simulink model "HANcoder_E407_GTSync_v5"  (R2018b)
settings: Solver=FixedStepDiscrete  StartTime=0.0  StopTime=1  FixedStep=0.01  RelTol=1e-3
PreLoadFcn:
  | librarySetup
  | eval([bdroot,'_startup']) %Calling [modelName]_startup.m
values from neighbouring files (symbols this model uses):
  basic_cycle_duration = TM_Reset_Board + COMP_duration    (= 170)    [HANcoder_E407_GTSync_v5_startup.m]
  comm_delay_estimation1 = round(comm_delay_measured*hardware_granularity/frequency_IRQ)    [HANcoder_E407_GTSync_v5_startup.m]
  comm_delay_estimation2 = round(comm_delay_measured*hardware_granularity/frequency_IRQ)    [HANcoder_E407_GTSync_v5_startup.m]
  COMM_Period = 25    [HANcoder_E407_GTSync_v5_startup.m]
  COMM_Phase1 = floor(COMM_Period/5)    [HANcoder_E407_GTSync_v5_startup.m]
  COMM_Phase2 = floor(4*COMM_Period/5)    [HANcoder_E407_GTSync_v5_startup.m]
  frequency_IRQ = 100    [HANcoder_E407_GTSync_v5_startup.m]
  HANtuneOverride = Simulink.Parameter    [HANcoder_E407_GTSync_v5_startup.m]
  idle_time_init = basic_cycle_duration*matrix_rows    (= 340)    [HANcoder_E407_GTSync_v5_startup.m]
  LED_ticks_toggle = 10000    [HANcoder_E407_GTSync_v5_startup.m]
  Master_Role = 1    [HANcoder_E407_GTSync_v5_startup.m]
  matrix_rows = 2    [HANcoder_E407_GTSync_v5_startup.m]
  MEX_Flag = 0    [HANcoder_E407_GTSync_v5_startup.m]
  Slave_Role = 2    [HANcoder_E407_GTSync_v5_startup.m]
  Sync_ID = 1    [HANcoder_E407_GTSync_v5_startup.m]
  TM_Check_Sync = TM_COMM_Sync   + COMM_duration    (= 30)    [HANcoder_E407_GTSync_v5_startup.m]
  TM_Check_TOuts = TM_Count_Vote3 + COMP_duration    (= 150)    [HANcoder_E407_GTSync_v5_startup.m]
  TM_Check_Vote1 = TM_COMM_Vote1  + COMM_duration    (= 70)    [HANcoder_E407_GTSync_v5_startup.m]
  TM_Check_Vote2 = TM_COMM_Vote2  + COMM_duration    (= 105)    [HANcoder_E407_GTSync_v5_startup.m]
  TM_Check_Vote3 = TM_COMM_Vote3  + COMM_duration    (= 140)    [HANcoder_E407_GTSync_v5_startup.m]
  TM_COMM_Sync = basic_cycle_start    (= 5)    [HANcoder_E407_GTSync_v5_startup.m]
  TM_COMM_Vote1 = TM_Vote_Dec    + COMP_duration    (= 45)    [HANcoder_E407_GTSync_v5_startup.m]
  TM_COMM_Vote2 = TM_Count_Vote1 + COMP_duration    (= 80)    [HANcoder_E407_GTSync_v5_startup.m]
  TM_COMM_Vote3 = TM_Count_Vote2 + COMP_duration    (= 115)    [HANcoder_E407_GTSync_v5_startup.m]
  TM_Count_Vote1 = TM_Check_Vote1 + COMP_duration    (= 75)    [HANcoder_E407_GTSync_v5_startup.m]
  TM_Count_Vote2 = TM_Check_Vote2 + COMP_duration    (= 110)    [HANcoder_E407_GTSync_v5_startup.m]
  TM_Count_Vote3 = TM_Check_Vote3 + COMP_duration    (= 145)    [HANcoder_E407_GTSync_v5_startup.m]
  TM_New_Master = TM_Check_TOuts + COMP_duration    (= 155)    [HANcoder_E407_GTSync_v5_startup.m]
  TM_Reset_Board = TM_Reset_Var   + COMP_duration    (= 165)    [HANcoder_E407_GTSync_v5_startup.m]
  TM_Reset_Var = TM_New_Master  + COMP_duration    (= 160)    [HANcoder_E407_GTSync_v5_startup.m]
  TM_Update_LT = TM_Check_Sync  + COMP_duration    (= 35)    [HANcoder_E407_GTSync_v5_startup.m]
  TM_Vote_Dec = TM_Update_LT   + COMP_duration    (= 40)    [HANcoder_E407_GTSync_v5_startup.m]
  Toggle_Flag = 1    [HANcoder_E407_GTSync_v5_startup.m]
  Vote1_ID = 12    [HANcoder_E407_GTSync_v5_startup.m]
  Vote2_ID = 22    [HANcoder_E407_GTSync_v5_startup.m]
  Vote3_ID = 32    [HANcoder_E407_GTSync_v5_startup.m]
undefined symbols (not defined in the file or in its folder): A0, A1, A2, A3, CON2
libraries: HANcoder_STM32_Target x25, hdlsllib x21, simulink x3, simulink_extras x1
(part 4 of 7)

== system HANcoder_E407_GTSync_v5/HANcoder STM32 Target - E407-STM32 algorithm/Global Ticks Increment/CAN Management/Matrix Cycle Manager/Matrix_Cycle_Observation_DEBUG ==
  Data Store Read : DataStoreRead  DataStoreName=Master_ID
  Data Store Read1 : DataStoreRead  DataStoreName=Role_ID
  Data Store Read10 : DataStoreRead  DataStoreName=time_difference_vote3
  Data Store Read11 : DataStoreRead  DataStoreName=sync_processed
  Data Store Read12 : DataStoreRead  DataStoreName=Rx_State_CAN1
  Data Store Read13 : DataStoreRead  DataStoreName=New_Msg_Ready_CAN1
  Data Store Read2 : DataStoreRead  DataStoreName=received_LT  DataStoreElements=received_LT.Local_Time_Board_1#received_LT.Local_Time_Board_2#received_LT.Local_Time_Board_3
  Data Store Read3 : DataStoreRead  DataStoreName=votes  DataStoreElements=votes.First_Board#votes.Second_Board#votes.Third_Board
  Data Store Read4 : DataStoreRead  DataStoreName=Board1_error_counter
  Data Store Read5 : DataStoreRead  DataStoreName=Board2_error_counter
  Data Store Read6 : DataStoreRead  DataStoreName=Board3_error_counter
  Data Store Read7 : DataStoreRead  DataStoreName=time_difference_sync
  Data Store Read8 : DataStoreRead  DataStoreName=time_difference_vote1
  Data Store Read9 : DataStoreRead  DataStoreName=time_difference_vote2
  Terminator{,1..17} (18 alike) : Terminator
  wires:
  Data Store Read1/1 -> Terminator/1  "Role_ID_DEBUG"
  Data Store Read/1 -> Terminator1/1  "Master_ID_DEBUG"
  Data Store Read2/1 -> Terminator2/1  "received_LT_Board_1_DEBUG"
  Data Store Read2/2 -> Terminator3/1  "received_LT_Board_2_DEBUG"
  Data Store Read2/3 -> Terminator4/1  "received_LT_Board_3_DEBUG"
  Data Store Read3/1 -> Terminator5/1  "votes_Board_1_DEBUG"
  Data Store Read3/2 -> Terminator6/1  "votes_Board_2_DEBUG"
  Data Store Read3/3 -> Terminator7/1  "votes_Board_3_DEBUG"
  Data Store Read4/1 -> Terminator8/1  "Board_1_error_counter_DEBUG"
  Data Store Read5/1 -> Terminator9/1  "Board_2_error_counter_DEBUG"
  Data Store Read6/1 -> Terminator10/1  "Board_3_error_counter_DEBUG"
  Data Store Read7/1 -> Terminator11/1  "time_difference_sync_DEBUG"
  Data Store Read8/1 -> Terminator12/1  "time_difference_vote_1_DEBUG"
  Data Store Read9/1 -> Terminator13/1  "time_difference_vote_2_DEBUG"
  Data Store Read10/1 -> Terminator14/1  "time_difference_vote_3_DEBUG"
  Data Store Read11/1 -> Terminator15/1  "sync_processed_s"
  Data Store Read12/1 -> Terminator16/1  "rx_state_s"
  Data Store Read13/1 -> Terminator17/1  "new_msg_ready_s"

== system HANcoder_E407_GTSync_v5/HANcoder STM32 Target - E407-STM32 algorithm/Global Ticks Increment/CAN1 Recieve/CAN receive/Enabled Subsystem ==
  In1 : Inport
  In2 : Inport  Port=2
  In3 : Inport  Port=3
  In4 : Inport  Port=4
  In5 : Inport  Port=5
  In6 : Inport  Port=6
  In7 : Inport  Port=7
  In8 : Inport  Port=8
  Enable : EnablePort
  Out1 : Outport
  Out2 : Outport  Port=2
  Out3 : Outport  Port=3
  Out4 : Outport  Port=4
  Out5 : Outport  Port=5
  Out6 : Outport  Port=6
  Out7 : Outport  Port=7
  Out8 : Outport  Port=8
  wires:
  In8/1 -> Out8/1
  In7/1 -> Out7/1
  In6/1 -> Out6/1
  In5/1 -> Out5/1
  In4/1 -> Out4/1
  In3/1 -> Out3/1
  In2/1 -> Out2/1
  In1/1 -> Out1/1

== system HANcoder_E407_GTSync_v5/HANcoder STM32 Target - E407-STM32 algorithm/Global Ticks Increment/CAN1 Recieve/RxID_CAN/Sync_ID_CAN ==
  Enable : EnablePort
  CAN receive : Subsystem  Tag=HANcoder_TARGET_STM32_E407  AncestorBlock=HANcoder_STM32_Target/STM32-E407/CAN/CAN/CAN receive  mask(CAN receive){canBus=CAN 1, outputNumber=8, dataType=uint8, byteOrder=off, tsamp=-1}
      mask prompts: canBus "CAN channel"; outputNumber "Output ports"; dataType "Output datatype"; byteOrder "Byte order: Checked = MSB first, unchecked = LSB first."; tsamp "Sample time"
      mask help:
      | Function
      | ==========
      | Receive the newest message from the specified CAN channel.
      |
      | Parameters
      | ==========
      | CAN channel:             The CAN channel to send the message on.
      | Output ports:             The amount of output ports
      | Output datatype:       The datatype of the output ports
      | Byte order:                 Select MSB or LSB first
      | Sample time:              -1 or divisible by base sample time [seconds]
      |
      | Input
      | ==========
      | Port 1:                       CAN ID(uint32) in hexadecimal ie: hex2dec('0a')
      |
      | Output
      | ==========
      | Port 1:                       Checks for new message(int8)
      | Port 2..9                     Message data
      mask init:
      | sfcn_can_receive_mcb(canBus, outputNumber, dataType, byteOrder)
      settings: MoveFcn=drawLogos
      mask Help: web('sfcn_can_receive.html');
      mask TypeOptions canBus: CAN 1 | CAN 2
      mask TypeOptions dataType: int8 | uint8 | int16 | uint16 | int32 | uint32 | boolean
      mask Display:
      | fprintf('Receive on\nCAN %x', canBus);
      | port_label('output', 1, 'new');
      | port_label('input', 1, 'ID');patch([135 141 141],[8 14 2],[1 0 0]);patch([143 143 149],[14 2 8],[0 0 0.35]);
  Constant : Constant  Value=Sync_ID  OutDataTypeStr=uint32
  CAN_new : Outport  OutputWhenDisabled=reset  InitialOutput=0
  Out2 : Outport  Port=2  OutputWhenDisabled=reset  InitialOutput=0
  Out3 : Outport  Port=3  OutputWhenDisabled=reset  InitialOutput=0
  Out4 : Outport  Port=4  OutputWhenDisabled=reset  InitialOutput=0
  Out5 : Outport  Port=5  OutputWhenDisabled=reset  InitialOutput=0
  Out6 : Outport  Port=6  OutputWhenDisabled=reset  InitialOutput=0
  Out7 : Outport  Port=7  OutputWhenDisabled=reset  InitialOutput=0
  Out8 : Outport  Port=8  OutputWhenDisabled=reset  InitialOutput=0
  Out9 : Outport  Port=9  OutputWhenDisabled=reset  InitialOutput=0
  wires:
  CAN receive/1(Out1) -> CAN_new/1
  CAN receive/8(Out8) -> Out8/1
  CAN receive/3(Out3) -> Out3/1
  Constant/1 -> CAN receive/1(In1)
  CAN receive/2(Out2) -> Out2/1
  CAN receive/6(Out6) -> Out6/1
  CAN receive/7(Out7) -> Out7/1
  CAN receive/4(Out4) -> Out4/1
  CAN receive/5(Out5) -> Out5/1
  CAN receive/9(Out9) -> Out9/1

== system HANcoder_E407_GTSync_v5/HANcoder STM32 Target - E407-STM32 algorithm/Global Ticks Increment/CAN1 Recieve/RxID_CAN/Vote1_ID_CAN ==
  Enable : EnablePort
  CAN receive : Subsystem  Tag=HANcoder_TARGET_STM32_E407  AncestorBlock=HANcoder_STM32_Target/STM32-E407/CAN/CAN/CAN receive  mask(CAN receive){canBus=CAN 1, outputNumber=8, dataType=uint8, byteOrder=off, tsamp=-1}
      mask prompts: canBus "CAN channel"; outputNumber "Output ports"; dataType "Output datatype"; byteOrder "Byte order: Checked = MSB first, unchecked = LSB first."; tsamp "Sample time"
      mask help:
      | Function
      | ==========
      | Receive the newest message from the specified CAN channel.
      |
      | Parameters
      | ==========
      | CAN channel:             The CAN channel to send the message on.
      | Output ports:             The amount of output ports
      | Output datatype:       The datatype of the output ports
      | Byte order:                 Select MSB or LSB first
      | Sample time:              -1 or divisible by base sample time [seconds]
      |
      | Input
      | ==========
      | Port 1:                       CAN ID(uint32) in hexadecimal ie: hex2dec('0a')
      |
      | Output
      | ==========
      | Port 1:                       Checks for new message(int8)
      | Port 2..9                     Message data
      mask init:
      | sfcn_can_receive_mcb(canBus, outputNumber, dataType, byteOrder)
      settings: MoveFcn=drawLogos
      mask Help: web('sfcn_can_receive.html');
      mask TypeOptions canBus: CAN 1 | CAN 2
      mask TypeOptions dataType: int8 | uint8 | int16 | uint16 | int32 | uint32 | boolean
      mask Display:
      | fprintf('Receive on\nCAN %x', canBus);
      | port_label('output', 1, 'new');
      | port_label('input', 1, 'ID');patch([135 141 141],[8 14 2],[1 0 0]);patch([143 143 149],[14 2 8],[0 0 0.35]);
  Constant : Constant  Value=Vote1_ID  OutDataTypeStr=uint32
  CAN_new : Outport  OutputWhenDisabled=reset  InitialOutput=0
  Out2 : Outport  Port=2  OutputWhenDisabled=reset  InitialOutput=0
  Out3 : Outport  Port=3  OutputWhenDisabled=reset  InitialOutput=0
  Out4 : Outport  Port=4  OutputWhenDisabled=reset  InitialOutput=0
  Out5 : Outport  Port=5  OutputWhenDisabled=reset  InitialOutput=0
  Out6 : Outport  Port=6  OutputWhenDisabled=reset  InitialOutput=0
  Out7 : Outport  Port=7  OutputWhenDisabled=reset  InitialOutput=0
  Out8 : Outport  Port=8  OutputWhenDisabled=reset  InitialOutput=0
  Out9 : Outport  Port=9  OutputWhenDisabled=reset  InitialOutput=0
  wires:
  CAN receive/9(Out9) -> Out9/1
  CAN receive/5(Out5) -> Out5/1
  CAN receive/4(Out4) -> Out4/1
  CAN receive/7(Out7) -> Out7/1
  CAN receive/6(Out6) -> Out6/1
  CAN receive/2(Out2) -> Out2/1
  Constant/1 -> CAN receive/1(In1)
  CAN receive/3(Out3) -> Out3/1
  CAN receive/8(Out8) -> Out8/1
  CAN receive/1(Out1) -> CAN_new/1

== system HANcoder_E407_GTSync_v5/HANcoder STM32 Target - E407-STM32 algorithm/Global Ticks Increment/CAN1 Recieve/RxID_CAN/Vote2_ID_CAN ==
  Enable : EnablePort
  CAN receive : Subsystem  Tag=HANcoder_TARGET_STM32_E407  AncestorBlock=HANcoder_STM32_Target/STM32-E407/CAN/CAN/CAN receive  mask(CAN receive){canBus=CAN 1, outputNumber=8, dataType=uint8, byteOrder=off, tsamp=-1}
      mask prompts: canBus "CAN channel"; outputNumber "Output ports"; dataType "Output datatype"; byteOrder "Byte order: Checked = MSB first, unchecked = LSB first."; tsamp "Sample time"
      mask help:
      | Function
      | ==========
      | Receive the newest message from the specified CAN channel.
      |
      | Parameters
      | ==========
      | CAN channel:             The CAN channel to send the message on.
      | Output ports:             The amount of output ports
      | Output datatype:       The datatype of the output ports
      | Byte order:                 Select MSB or LSB first
      | Sample time:              -1 or divisible by base sample time [seconds]
      |
      | Input
      | ==========
      | Port 1:                       CAN ID(uint32) in hexadecimal ie: hex2dec('0a')
      |
      | Output
      | ==========
      | Port 1:                       Checks for new message(int8)
      | Port 2..9                     Message data
      mask init:
      | sfcn_can_receive_mcb(canBus, outputNumber, dataType, byteOrder)
      settings: MoveFcn=drawLogos
      mask Help: web('sfcn_can_receive.html');
      mask TypeOptions canBus: CAN 1 | CAN 2
      mask TypeOptions dataType: int8 | uint8 | int16 | uint16 | int32 | uint32 | boolean
      mask Display:
      | fprintf('Receive on\nCAN %x', canBus);
      | port_label('output', 1, 'new');
      | port_label('input', 1, 'ID');patch([135 141 141],[8 14 2],[1 0 0]);patch([143 143 149],[14 2 8],[0 0 0.35]);
  Constant : Constant  Value=Vote2_ID  OutDataTypeStr=uint32
  CAN_new : Outport  OutputWhenDisabled=reset  InitialOutput=0
  Out2 : Outport  Port=2  OutputWhenDisabled=reset  InitialOutput=0
  Out3 : Outport  Port=3  OutputWhenDisabled=reset  InitialOutput=0
  Out4 : Outport  Port=4  OutputWhenDisabled=reset  InitialOutput=0
  Out5 : Outport  Port=5  OutputWhenDisabled=reset  InitialOutput=0
  Out6 : Outport  Port=6  OutputWhenDisabled=reset  InitialOutput=0
  Out7 : Outport  Port=7  OutputWhenDisabled=reset  InitialOutput=0
  Out8 : Outport  Port=8  OutputWhenDisabled=reset  InitialOutput=0
  Out9 : Outport  Port=9  OutputWhenDisabled=reset  InitialOutput=0
  wires:
  CAN receive/1(Out1) -> CAN_new/1
  CAN receive/8(Out8) -> Out8/1
  CAN receive/3(Out3) -> Out3/1
  Constant/1 -> CAN receive/1(In1)
  CAN receive/2(Out2) -> Out2/1
  CAN receive/6(Out6) -> Out6/1
  CAN receive/7(Out7) -> Out7/1
  CAN receive/4(Out4) -> Out4/1
  CAN receive/5(Out5) -> Out5/1
  CAN receive/9(Out9) -> Out9/1

== system HANcoder_E407_GTSync_v5/HANcoder STM32 Target - E407-STM32 algorithm/Global Ticks Increment/CAN1 Recieve/RxID_CAN/Vote3_ID_CAN ==
  Enable : EnablePort
  CAN receive : Subsystem  Tag=HANcoder_TARGET_STM32_E407  AncestorBlock=HANcoder_STM32_Target/STM32-E407/CAN/CAN/CAN receive  mask(CAN receive){canBus=CAN 1, outputNumber=8, dataType=uint8, byteOrder=off, tsamp=-1}
      mask prompts: canBus "CAN channel"; outputNumber "Output ports"; dataType "Output datatype"; byteOrder "Byte order: Checked = MSB first, unchecked = LSB first."; tsamp "Sample time"
      mask help:
      | Function
      | ==========
      | Receive the newest message from the specified CAN channel.
      |
      | Parameters
      | ==========
      | CAN channel:             The CAN channel to send the message on.
      | Output ports:             The amount of output ports
      | Output datatype:       The datatype of the output ports
      | Byte order:                 Select MSB or LSB first
      | Sample time:              -1 or divisible by base sample time [seconds]
      |
      | Input
      | ==========
      | Port 1:                       CAN ID(uint32) in hexadecimal ie: hex2dec('0a')
      |
      | Output
      | ==========
      | Port 1:                       Checks for new message(int8)
      | Port 2..9                     Message data
      mask init:
      | sfcn_can_receive_mcb(canBus, outputNumber, dataType, byteOrder)
      settings: MoveFcn=drawLogos
      mask Help: web('sfcn_can_receive.html');
      mask TypeOptions canBus: CAN 1 | CAN 2
      mask TypeOptions dataType: int8 | uint8 | int16 | uint16 | int32 | uint32 | boolean
      mask Display:
      | fprintf('Receive on\nCAN %x', canBus);
      | port_label('output', 1, 'new');
      | port_label('input', 1, 'ID');patch([135 141 141],[8 14 2],[1 0 0]);patch([143 143 149],[14 2 8],[0 0 0.35]);
  Constant : Constant  Value=Vote3_ID  OutDataTypeStr=uint32
  CAN_new : Outport  OutputWhenDisabled=reset  InitialOutput=0
  Out2 : Outport  Port=2  OutputWhenDisabled=reset  InitialOutput=0
  Out3 : Outport  Port=3  OutputWhenDisabled=reset  InitialOutput=0
  Out4 : Outport  Port=4  OutputWhenDisabled=reset  InitialOutput=0
  Out5 : Outport  Port=5  OutputWhenDisabled=reset  InitialOutput=0
  Out6 : Outport  Port=6  OutputWhenDisabled=reset  InitialOutput=0
  Out7 : Outport  Port=7  OutputWhenDisabled=reset  InitialOutput=0
  Out8 : Outport  Port=8  OutputWhenDisabled=reset  InitialOutput=0
  Out9 : Outport  Port=9  OutputWhenDisabled=reset  InitialOutput=0
  wires:
  CAN receive/9(Out9) -> Out9/1
  CAN receive/5(Out5) -> Out5/1
  CAN receive/4(Out4) -> Out4/1
  CAN receive/7(Out7) -> Out7/1
  CAN receive/6(Out6) -> Out6/1
  CAN receive/2(Out2) -> Out2/1
  Constant/1 -> CAN receive/1(In1)
  CAN receive/3(Out3) -> Out3/1
  CAN receive/8(Out8) -> Out8/1
  CAN receive/1(Out1) -> CAN_new/1

== system HANcoder_E407_GTSync_v5/HANcoder STM32 Target - E407-STM32 algorithm/Global Ticks Increment/CAN2 Recieve/CAN receive/Enabled Subsystem ==
  In1 : Inport
  In2 : Inport  Port=2
  In3 : Inport  Port=3
  In4 : Inport  Port=4
  In5 : Inport  Port=5
  In6 : Inport  Port=6
  In7 : Inport  Port=7
  In8 : Inport  Port=8
  Enable : EnablePort
  Out1 : Outport
  Out2 : Outport  Port=2
  Out3 : Outport  Port=3
  Out4 : Outport  Port=4
  Out5 : Outport  Port=5
  Out6 : Outport  Port=6
  Out7 : Outport  Port=7
  Out8 : Outport  Port=8
  wires:
  In8/1 -> Out8/1
  In7/1 -> Out7/1
  In6/1 -> Out6/1
  In5/1 -> Out5/1
  In4/1 -> Out4/1
  In3/1 -> Out3/1
  In2/1 -> Out2/1
  In1/1 -> Out1/1

== system HANcoder_E407_GTSync_v5/HANcoder STM32 Target - E407-STM32 algorithm/Global Ticks Increment/CAN2 Recieve/RxID_CAN/Sync_ID_CAN ==
  Enable : EnablePort
  CAN receive : Subsystem  Tag=HANcoder_TARGET_STM32_E407  AncestorBlock=HANcoder_STM32_Target/STM32-E407/CAN/CAN/CAN receive  mask(CAN receive){canBus=CAN 2, outputNumber=8, dataType=uint8, byteOrder=off, tsamp=-1}
      mask prompts: canBus "CAN channel"; outputNumber "Output ports"; dataType "Output datatype"; byteOrder "Byte order: Checked = MSB first, unchecked = LSB first."; tsamp "Sample time"
      mask help:
      | Function
      | ==========
      | Receive the newest message from the specified CAN channel.
      |
      | Parameters
      | ==========
      | CAN channel:             The CAN channel to send the message on.
      | Output ports:             The amount of output ports
      | Output datatype:       The datatype of the output ports
      | Byte order:                 Select MSB or LSB first
      | Sample time:              -1 or divisible by base sample time [seconds]
      |
      | Input
      | ==========
      | Port 1:                       CAN ID(uint32) in hexadecimal ie: hex2dec('0a')
      |
      | Output
      | ==========
      | Port 1:                       Checks for new message(int8)
      | Port 2..9                     Message data
      mask init:
      | sfcn_can_receive_mcb(canBus, outputNumber, dataType, byteOrder)
      settings: MoveFcn=drawLogos
      mask Help: web('sfcn_can_receive.html');
      mask TypeOptions canBus: CAN 1 | CAN 2
      mask TypeOptions dataType: int8 | uint8 | int16 | uint16 | int32 | uint32 | boolean
      mask Display:
      | fprintf('Receive on\nCAN %x', canBus);
      | port_label('output', 1, 'new');
      | port_label('input', 1, 'ID');patch([135 141 141],[8 14 2],[1 0 0]);patch([143 143 149],[14 2 8],[0 0 0.35]);
  Constant : Constant  Value=Sync_ID  OutDataTypeStr=uint32
  CAN_new : Outport  OutputWhenDisabled=reset  InitialOutput=0
  Out2 : Outport  Port=2  OutputWhenDisabled=reset  InitialOutput=0
  Out3 : Outport  Port=3  OutputWhenDisabled=reset  InitialOutput=0
  Out4 : Outport  Port=4  OutputWhenDisabled=reset  InitialOutput=0
  Out5 : Outport  Port=5  OutputWhenDisabled=reset  InitialOutput=0
  Out6 : Outport  Port=6  OutputWhenDisabled=reset  InitialOutput=0
  Out7 : Outport  Port=7  OutputWhenDisabled=reset  InitialOutput=0
  Out8 : Outport  Port=8  OutputWhenDisabled=reset  InitialOutput=0
  Out9 : Outport  Port=9  OutputWhenDisabled=reset  InitialOutput=0
  wires:
  CAN receive/9(Out9) -> Out9/1
  CAN receive/5(Out5) -> Out5/1
  CAN receive/4(Out4) -> Out4/1
  CAN receive/7(Out7) -> Out7/1
  CAN receive/6(Out6) -> Out6/1
  CAN receive/2(Out2) -> Out2/1
  Constant/1 -> CAN receive/1(In1)
  CAN receive/3(Out3) -> Out3/1
  CAN receive/8(Out8) -> Out8/1
  CAN receive/1(Out1) -> CAN_new/1

== system HANcoder_E407_GTSync_v5/HANcoder STM32 Target - E407-STM32 algorithm/Global Ticks Increment/CAN2 Recieve/RxID_CAN/Vote1_ID_CAN ==
  Enable : EnablePort
  CAN receive : Subsystem  Tag=HANcoder_TARGET_STM32_E407  AncestorBlock=HANcoder_STM32_Target/STM32-E407/CAN/CAN/CAN receive  mask(CAN receive){canBus=CAN 2, outputNumber=8, dataType=uint8, byteOrder=off, tsamp=-1}
      mask prompts: canBus "CAN channel"; outputNumber "Output ports"; dataType "Output datatype"; byteOrder "Byte order: Checked = MSB first, unchecked = LSB first."; tsamp "Sample time"
      mask help:
      | Function
      | ==========
      | Receive the newest message from the specified CAN channel.
      |
      | Parameters
      | ==========
      | CAN channel:             The CAN channel to send the message on.
      | Output ports:             The amount of output ports
      | Output datatype:       The datatype of the output ports
      | Byte order:                 Select MSB or LSB first
      | Sample time:              -1 or divisible by base sample time [seconds]
      |
      | Input
      | ==========
      | Port 1:                       CAN ID(uint32) in hexadecimal ie: hex2dec('0a')
      |
      | Output
      | ==========
      | Port 1:                       Checks for new message(int8)
      | Port 2..9                     Message data
      mask init:
      | sfcn_can_receive_mcb(canBus, outputNumber, dataType, byteOrder)
      settings: MoveFcn=drawLogos
      mask Help: web('sfcn_can_receive.html');
      mask TypeOptions canBus: CAN 1 | CAN 2
      mask TypeOptions dataType: int8 | uint8 | int16 | uint16 | int32 | uint32 | boolean
      mask Display:
      | fprintf('Receive on\nCAN %x', canBus);
      | port_label('output', 1, 'new');
      | port_label('input', 1, 'ID');patch([135 141 141],[8 14 2],[1 0 0]);patch([143 143 149],[14 2 8],[0 0 0.35]);
  Constant : Constant  Value=Vote1_ID  OutDataTypeStr=uint32
  CAN_new : Outport  OutputWhenDisabled=reset  InitialOutput=0
  Out2 : Outport  Port=2  OutputWhenDisabled=reset  InitialOutput=0
  Out3 : Outport  Port=3  OutputWhenDisabled=reset  InitialOutput=0
  Out4 : Outport  Port=4  OutputWhenDisabled=reset  InitialOutput=0
  Out5 : Outport  Port=5  OutputWhenDisabled=reset  InitialOutput=0
  Out6 : Outport  Port=6  OutputWhenDisabled=reset  InitialOutput=0
  Out7 : Outport  Port=7  OutputWhenDisabled=reset  InitialOutput=0
  Out8 : Outport  Port=8  OutputWhenDisabled=reset  InitialOutput=0
  Out9 : Outport  Port=9  OutputWhenDisabled=reset  InitialOutput=0
  wires:
  CAN receive/1(Out1) -> CAN_new/1
  CAN receive/8(Out8) -> Out8/1
  CAN receive/3(Out3) -> Out3/1
  Constant/1 -> CAN receive/1(In1)
  CAN receive/2(Out2) -> Out2/1
  CAN receive/6(Out6) -> Out6/1
  CAN receive/7(Out7) -> Out7/1
  CAN receive/4(Out4) -> Out4/1
  CAN receive/5(Out5) -> Out5/1
  CAN receive/9(Out9) -> Out9/1

== system HANcoder_E407_GTSync_v5/HANcoder STM32 Target - E407-STM32 algorithm/Global Ticks Increment/CAN2 Recieve/RxID_CAN/Vote2_ID_CAN ==
  Enable : EnablePort
  CAN receive : Subsystem  Tag=HANcoder_TARGET_STM32_E407  AncestorBlock=HANcoder_STM32_Target/STM32-E407/CAN/CAN/CAN receive  mask(CAN receive){canBus=CAN 2, outputNumber=8, dataType=uint8, byteOrder=off, tsamp=-1}
      mask prompts: canBus "CAN channel"; outputNumber "Output ports"; dataType "Output datatype"; byteOrder "Byte order: Checked = MSB first, unchecked = LSB first."; tsamp "Sample time"
      mask help:
      | Function
      | ==========
      | Receive the newest message from the specified CAN channel.
      |
      | Parameters
      | ==========
      | CAN channel:             The CAN channel to send the message on.
      | Output ports:             The amount of output ports
      | Output datatype:       The datatype of the output ports
      | Byte order:                 Select MSB or LSB first
      | Sample time:              -1 or divisible by base sample time [seconds]
      |
      | Input
      | ==========
      | Port 1:                       CAN ID(uint32) in hexadecimal ie: hex2dec('0a')
      |
      | Output
      | ==========
      | Port 1:                       Checks for new message(int8)
      | Port 2..9                     Message data
      mask init:
      | sfcn_can_receive_mcb(canBus, outputNumber, dataType, byteOrder)
      settings: MoveFcn=drawLogos
      mask Help: web('sfcn_can_receive.html');
      mask TypeOptions canBus: CAN 1 | CAN 2
      mask TypeOptions dataType: int8 | uint8 | int16 | uint16 | int32 | uint32 | boolean
      mask Display:
      | fprintf('Receive on\nCAN %x', canBus);
      | port_label('output', 1, 'new');
      | port_label('input', 1, 'ID');patch([135 141 141],[8 14 2],[1 0 0]);patch([143 143 149],[14 2 8],[0 0 0.35]);
  Constant : Constant  Value=Vote2_ID  OutDataTypeStr=uint32
  CAN_new : Outport  OutputWhenDisabled=reset  InitialOutput=0
  Out2 : Outport  Port=2  OutputWhenDisabled=reset  InitialOutput=0
  Out3 : Outport  Port=3  OutputWhenDisabled=reset  InitialOutput=0
  Out4 : Outport  Port=4  OutputWhenDisabled=reset  InitialOutput=0
  Out5 : Outport  Port=5  OutputWhenDisabled=reset  InitialOutput=0
  Out6 : Outport  Port=6  OutputWhenDisabled=reset  InitialOutput=0
  Out7 : Outport  Port=7  OutputWhenDisabled=reset  InitialOutput=0
  Out8 : Outport  Port=8  OutputWhenDisabled=reset  InitialOutput=0
  Out9 : Outport  Port=9  OutputWhenDisabled=reset  InitialOutput=0
  wires:
  CAN receive/9(Out9) -> Out9/1
  CAN receive/5(Out5) -> Out5/1
  CAN receive/4(Out4) -> Out4/1
  CAN receive/7(Out7) -> Out7/1
  CAN receive/6(Out6) -> Out6/1
  CAN receive/2(Out2) -> Out2/1
  Constant/1 -> CAN receive/1(In1)
  CAN receive/3(Out3) -> Out3/1
  CAN receive/8(Out8) -> Out8/1
  CAN receive/1(Out1) -> CAN_new/1

== system HANcoder_E407_GTSync_v5/HANcoder STM32 Target - E407-STM32 algorithm/Global Ticks Increment/CAN2 Recieve/RxID_CAN/Vote3_ID_CAN ==
  Enable : EnablePort
  CAN receive : Subsystem  Tag=HANcoder_TARGET_STM32_E407  AncestorBlock=HANcoder_STM32_Target/STM32-E407/CAN/CAN/CAN receive  mask(CAN receive){canBus=CAN 2, outputNumber=8, dataType=uint8, byteOrder=off, tsamp=-1}
      mask prompts: canBus "CAN channel"; outputNumber "Output ports"; dataType "Output datatype"; byteOrder "Byte order: Checked = MSB first, unchecked = LSB first."; tsamp "Sample time"
      mask help:
      | Function
      | ==========
      | Receive the newest message from the specified CAN channel.
      |
      | Parameters
      | ==========
      | CAN channel:             The CAN channel to send the message on.
      | Output ports:             The amount of output ports
      | Output datatype:       The datatype of the output ports
      | Byte order:                 Select MSB or LSB first
      | Sample time:              -1 or divisible by base sample time [seconds]
      |
      | Input
      | ==========
      | Port 1:                       CAN ID(uint32) in hexadecimal ie: hex2dec('0a')
      |
      | Output
      | ==========
      | Port 1:                       Checks for new message(int8)
      | Port 2..9                     Message data
      mask init:
      | sfcn_can_receive_mcb(canBus, outputNumber, dataType, byteOrder)
      settings: MoveFcn=drawLogos
      mask Help: web('sfcn_can_receive.html');
      mask TypeOptions canBus: CAN 1 | CAN 2
      mask TypeOptions dataType: int8 | uint8 | int16 | uint16 | int32 | uint32 | boolean
      mask Display:
      | fprintf('Receive on\nCAN %x', canBus);
      | port_label('output', 1, 'new');
      | port_label('input', 1, 'ID');patch([135 141 141],[8 14 2],[1 0 0]);patch([143 143 149],[14 2 8],[0 0 0.35]);
  Constant : Constant  Value=Vote3_ID  OutDataTypeStr=uint32
  CAN_new : Outport  OutputWhenDisabled=reset  InitialOutput=0
  Out2 : Outport  Port=2  OutputWhenDisabled=reset  InitialOutput=0
  Out3 : Outport  Port=3  OutputWhenDisabled=reset  InitialOutput=0
  Out4 : Outport  Port=4  OutputWhenDisabled=reset  InitialOutput=0
  Out5 : Outport  Port=5  OutputWhenDisabled=reset  InitialOutput=0
  Out6 : Outport  Port=6  OutputWhenDisabled=reset  InitialOutput=0
  Out7 : Outport  Port=7  OutputWhenDisabled=reset  InitialOutput=0
  Out8 : Outport  Port=8  OutputWhenDisabled=reset  InitialOutput=0
  Out9 : Outport  Port=9  OutputWhenDisabled=reset  InitialOutput=0
  wires:
  CAN receive/1(Out1) -> CAN_new/1
  CAN receive/8(Out8) -> Out8/1
  CAN receive/3(Out3) -> Out3/1
  Constant/1 -> CAN receive/1(In1)
  CAN receive/2(Out2) -> Out2/1
  CAN receive/6(Out6) -> Out6/1
  CAN receive/7(Out7) -> Out7/1
  CAN receive/4(Out4) -> Out4/1
  CAN receive/5(Out5) -> Out5/1
  CAN receive/9(Out9) -> Out9/1

== system HANcoder_E407_GTSync_v5/HANcoder STM32 Target - E407-STM32 algorithm/Global Ticks Increment/CAN Management/Initialization/Delay/Initializaton_Observation_DEBUG ==
  Data Store Read : DataStoreRead  DataStoreName=Initialization_flag
  Data Store Read1 : DataStoreRead  DataStoreName=Delay_Counter
  Data Store Read2 : DataStoreRead  DataStoreName=New_Msg_Ready_CAN1
  Data Store Read3 : DataStoreRead  DataStoreName=Initialization_Timeout
  Data Store Read5 : DataStoreRead  DataStoreName=basic_cycle_count
  Terminator{,1..3,5} (5 alike) : Terminator
  wires:
  Data Store Read3/1 -> Terminator3/1  "initialization_timeout_DEBUG"
  Data Store Read1/1 -> Terminator1/1  "delay_counter_DEBUG"
  Data Store Read/1 -> Terminator/1  "initialization_flag_DEBUG"
  Data Store Read5/1 -> Terminator5/1  "basic_cycle_DEBUG"
  Data Store Read2/1 -> Terminator2/1  "New_Msg_Rx_DEBUG"

== system HANcoder_E407_GTSync_v5/HANcoder STM32 Target - E407-STM32 algorithm/Global Ticks Increment/CAN Management/Initialization/RoleID and Global Time init/Global Time Initialization Master ==
  note: Global Time Initialization
  Enable : EnablePort
  Board nr1 : Constant
  Data Store Write3 : DataStoreWrite  DataStoreName=Master_ID
  wires:
  Board nr1/1 -> Data Store Write3/1

== system HANcoder_E407_GTSync_v5/HANcoder STM32 Target - E407-STM32 algorithm/Global Ticks Increment/CAN Management/Initialization/RoleID and Global Time init/Global Time Initialization Slave ==
  note: Global Time Initialization
  Enable : EnablePort
  Bus Selector : BusSelector  OutputSignals=Buffer_1,Buffer_2,Buffer_3,Buffer_4,Buffer_5,Buffer_6,Buffer_7,Buffer_8
  Constant : Constant
  Data Store Read : DataStoreRead  DataStoreName=New_Msg_Ready_CAN1
  Data Store Read1 : DataStoreRead  DataStoreName=Msg_Rx_CAN1
  Data Store Read2 : DataStoreRead  DataStoreName=Msg_Rx_CAN2
  Data Store Write1 : DataStoreWrite  DataStoreName=Local_Ticks
  Data Store Write2 : DataStoreWrite  DataStoreName=basic_cycle_count
  Data Store Write3 : DataStoreWrite  DataStoreName=Master_ID
  Data Type Conversion{1..9} (9 alike) : DataTypeConversion  OutDataTypeStr=double
  Equal : RelationalOperator  Operator===  OutDataTypeStr=boolean  RndMeth=Simplest
  Switch : Switch  Criteria=u2 > Threshold
  Terminator{1..8} (8 alike) : Terminator
  UINT8 to UINT16 : Subsystem
  wires:
  Bus Selector/4 -> Data Store Write2/1, Data Type Conversion5/1  "<Buffer_4>"
  Data Store Read/1 -> Equal/1
  Constant/1 -> Equal/2
  Data Type Conversion7/1 -> Terminator3/1  "CAN1_received_message_2"
  Data Type Conversion1/1 -> Terminator8/1  "CAN1_received_local_time_1"
  Bus Selector/5 -> Data Type Conversion6/1  "<Buffer_5>"
  Data Type Conversion6/1 -> Terminator4/1  "CAN1_received_message_1"
  UINT8 to UINT16/1(Out1) -> Data Store Write1/1, Data Type Conversion2/1  "CAN1_received_local_time_update"
  Data Type Conversion8/1 -> Terminator6/1  "CAN1_received_message_3"
  Bus Selector/3 -> Data Type Conversion4/1, UINT8 to UINT16/2(In2)  "<Buffer_3>"
  Data Type Conversion4/1 -> Terminator2/1  "CAN1_received_local_time_2"
  Data Type Conversion5/1 -> Terminator1/1  "CAN1_received_basic_cycle"
  Bus Selector/8 -> Data Type Conversion9/1  "<Buffer_8>"
  Bus Selector/7 -> Data Type Conversion8/1  "<Buffer_7>"
  Bus Selector/6 -> Data Type Conversion7/1  "<Buffer_6>"
  Data Type Conversion2/1 -> Terminator5/1  "CAN1_received_local_time"
  Bus Selector/2 -> Data Type Conversion1/1, UINT8 to UINT16/1(In1)  "<Buffer_2>"
  Data Type Conversion9/1 -> Terminator7/1  "CAN1_received_message_4"
  Switch/1 -> Bus Selector/1
  Bus Selector/1 -> Data Type Conversion3/1  "<Buffer_1>"
  Data Type Conversion3/1 -> Data Store Write3/1  "CAN1_Message_Header_s"
  Equal/1 -> Switch/2
  Data Store Read1/1 -> Switch/1
  Data Store Read2/1 -> Switch/3

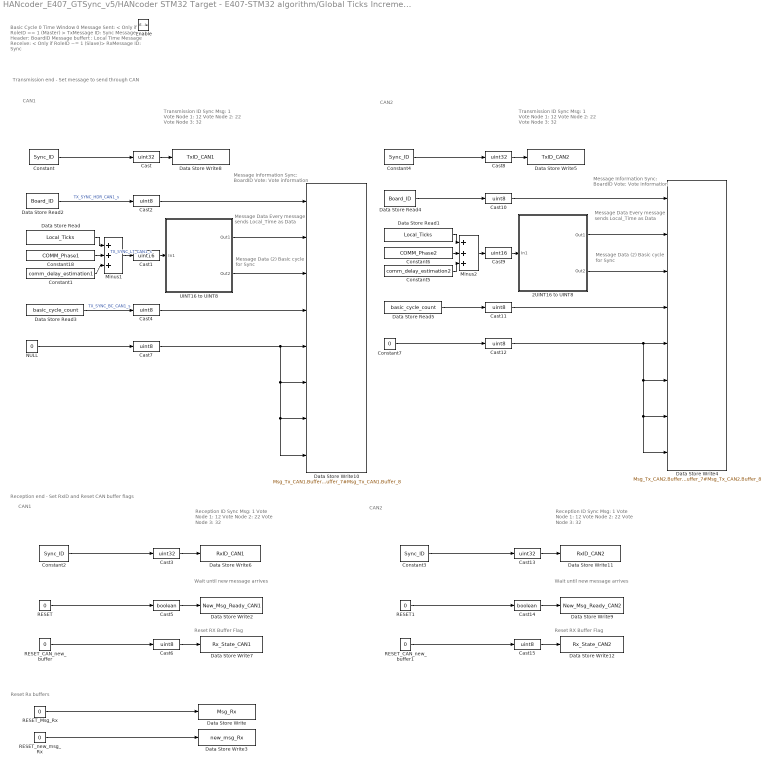
== system HANcoder_E407_GTSync_v5/HANcoder STM32 Target - E407-STM32 algorithm/Global Ticks Increment/CAN Management/Matrix Cycle Manager/COMM Task - Sync BC0/Sync Msg ==
  note: CAN2
  note: CAN1
  note: Transmission end - Set message to send through CAN
  note: CAN2
  note: CAN1
  note: Reception end - Set RxID and Reset CAN buffer flags
  note: Reset Rx buffers
  note: Wait until new message
      | arrives
  note: Message Data (2)
      |    Basic cycle for Sync
  note: Basic Cycle 0
      | Time Window 0
      | Message Sent: < Only if RoleID == 1 (Master) >
      | 	TxMessage ID: Sync
      | 	Message Header: BoardID
      | 	Message buffert : Local Time
      | Message Receive: < Only if RoleID ~= 1 (Slave)>
      | 	RxMessage ID: Sync
  note: Message Data
      |    Every message sends
      |    Local_Time as Data
  note: Transmission ID
      |    Sync Msg: 1
      |    Vote Node 1: 12
      |    Vote Node 2: 22
      |    Vote Node 3: 32
  note: Message Information
      |    Sync: BoardID
      |    Vote: Vote information
  note: Reception ID
      |    Sync Msg: 1
      |    Vote Node 1: 12
      |    Vote Node 2: 22
      |    Vote Node 3: 32
  note: Reset RX Buffer Flag
  note: Message Data (2)
      |    Basic cycle for Sync
  note: Message Data
      |    Every message sends
      |    Local_Time as Data
  note: Transmission ID
      |    Sync Msg: 1
      |    Vote Node 1: 12
      |    Vote Node 2: 22
      |    Vote Node 3: 32
  note: Message Information
      |    Sync: BoardID
      |    Vote: Vote information
  note: Wait until new message
      | arrives
  note: Reception ID
      |    Sync Msg: 1
      |    Vote Node 1: 12
      |    Vote Node 2: 22
      |    Vote Node 3: 32
  note: Reset RX Buffer Flag
  Enable : EnablePort
  2UINT16 to UINT8 : Subsystem
  Cast{,3,8,13} (4 alike) : DataTypeConversion  OutDataTypeStr=uint32
  Cast1 : DataTypeConversion  OutDataTypeStr=uint16
  Cast{2,4,6..7,10..12,15} (8 alike) : DataTypeConversion  OutDataTypeStr=uint8
  Cast14 : DataTypeConversion  OutDataTypeStr=boolean
  Cast5 : DataTypeConversion  OutDataTypeStr=boolean
  Cast9 : DataTypeConversion  OutDataTypeStr=uint16
  Constant{,2..4} (4 alike) : Constant  Value=Sync_ID
  Constant1 : Constant  Value=comm_delay_estimation1
  Constant18 : Constant  Value=COMM_Phase1
  Constant5 : Constant  Value=comm_delay_estimation2
  Constant6 : Constant  Value=COMM_Phase2
  Constant7 : Constant  Value=0  OutDataTypeStr=uint8
  Data Store Read : DataStoreRead  DataStoreName=Local_Ticks
  Data Store Read1 : DataStoreRead  DataStoreName=Local_Ticks
  Data Store Read2 : DataStoreRead  DataStoreName=Board_ID
  Data Store Read3 : DataStoreRead  DataStoreName=basic_cycle_count
  Data Store Read4 : DataStoreRead  DataStoreName=Board_ID
  Data Store Read5 : DataStoreRead  DataStoreName=basic_cycle_count
  Data Store Write : DataStoreWrite  DataStoreName=Msg_Rx
  Data Store Write10 : DataStoreWrite  DataStoreName=Msg_Tx_CAN1  DataStoreElements=Msg_Tx_CAN1.Buffer_1#Msg_Tx_CAN1.Buffer_2#Msg_Tx_CAN1.Buffer_3#Msg_Tx_CAN1.Buffer_4#Msg_Tx_CAN1.Buffer_5#Msg_Tx_CAN1.Buffer_6#Msg_Tx_CAN1.Buffer_7#Msg_Tx_CAN1.Buffer_8
  Data Store Write11 : DataStoreWrite  DataStoreName=RxID_CAN2
  Data Store Write12 : DataStoreWrite  DataStoreName=Rx_State_CAN2
  Data Store Write2 : DataStoreWrite  DataStoreName=New_Msg_Ready_CAN1
  Data Store Write3 : DataStoreWrite  DataStoreName=new_msg_Rx
  Data Store Write4 : DataStoreWrite  DataStoreName=Msg_Tx_CAN2  DataStoreElements=Msg_Tx_CAN2.Buffer_1#Msg_Tx_CAN2.Buffer_2#Msg_Tx_CAN2.Buffer_3#Msg_Tx_CAN2.Buffer_4#Msg_Tx_CAN2.Buffer_5#Msg_Tx_CAN2.Buffer_6#Msg_Tx_CAN2.Buffer_7#Msg_Tx_CAN2.Buffer_8
  Data Store Write5 : DataStoreWrite  DataStoreName=TxID_CAN2
  Data Store Write6 : DataStoreWrite  DataStoreName=RxID_CAN1
  Data Store Write7 : DataStoreWrite  DataStoreName=Rx_State_CAN1
  Data Store Write8 : DataStoreWrite  DataStoreName=TxID_CAN1
  Data Store Write9 : DataStoreWrite  DataStoreName=New_Msg_Ready_CAN2
  Minus1 : Sum  Inputs=+++
  Minus2 : Sum  Inputs=+++
  NULL : Constant  Value=0  OutDataTypeStr=uint8
  RESET : Constant  Value=0
  RESET1 : Constant  Value=0
  RESET_CAN_new_buffer : Constant  Value=0
  RESET_CAN_new_buffer1 : Constant  Value=0
  RESET_Msg_Rx : Constant  Value=0  OutDataTypeStr=Bus: demux_msg_buffer_type
  RESET_new_msg_Rx : Constant  Value=0  OutDataTypeStr=boolean
  UINT16 to UINT8 : Subsystem
  wires:
  Constant18/1 -> Minus1/2
  Minus1/1 -> Cast1/1  "TX_SYNC_LT_CAN1_s"
  Cast/1 -> Data Store Write8/1
  Data Store Read/1 -> Minus1/1
  Constant/1 -> Cast/1
  Cast3/1 -> Data Store Write6/1
  Constant2/1 -> Cast3/1
  Cast2/1 -> Data Store Write10/1
  Cast4/1 -> Data Store Write10/4
  Data Store Read3/1 -> Cast4/1  "TX_SYNC_BC_CAN1_s"
  Data Store Read2/1 -> Cast2/1  "TX_SYNC_HDR_CAN1_s"
  RESET/1 -> Cast5/1
  Cast5/1 -> Data Store Write2/1
  RESET_Msg_Rx/1 -> Data Store Write/1
  RESET_new_msg_Rx/1 -> Data Store Write3/1
  RESET_CAN_new_buffer/1 -> Cast6/1
  Cast6/1 -> Data Store Write7/1
  Constant1/1 -> Minus1/3
  Cast1/1 -> UINT16 to UINT8/1(In1)
  UINT16 to UINT8/2(Out2) -> Data Store Write10/3
  UINT16 to UINT8/1(Out1) -> Data Store Write10/2
  Cast7/1 -> Data Store Write10/8, Data Store Write10/7, Data Store Write10/6, Data Store Write10/5
  NULL/1 -> Cast7/1
  Constant7/1 -> Cast12/1
  Cast12/1 -> Data Store Write4/8, Data Store Write4/7, Data Store Write4/6, Data Store Write4/5
  2UINT16 to UINT8/1(Out1) -> Data Store Write4/2
  2UINT16 to UINT8/2(Out2) -> Data Store Write4/3
  Cast9/1 -> 2UINT16 to UINT8/1(In1)
  Constant5/1 -> Minus2/3
  Data Store Read4/1 -> Cast10/1
  Data Store Read5/1 -> Cast11/1
  Cast11/1 -> Data Store Write4/4
  Cast10/1 -> Data Store Write4/1
  Constant4/1 -> Cast8/1
  Data Store Read1/1 -> Minus2/1
  Cast8/1 -> Data Store Write5/1
  Minus2/1 -> Cast9/1
  Constant6/1 -> Minus2/2
  Cast15/1 -> Data Store Write12/1
  RESET_CAN_new_buffer1/1 -> Cast15/1
  Cast14/1 -> Data Store Write9/1
  RESET1/1 -> Cast14/1
  Constant3/1 -> Cast13/1
  Cast13/1 -> Data Store Write11/1

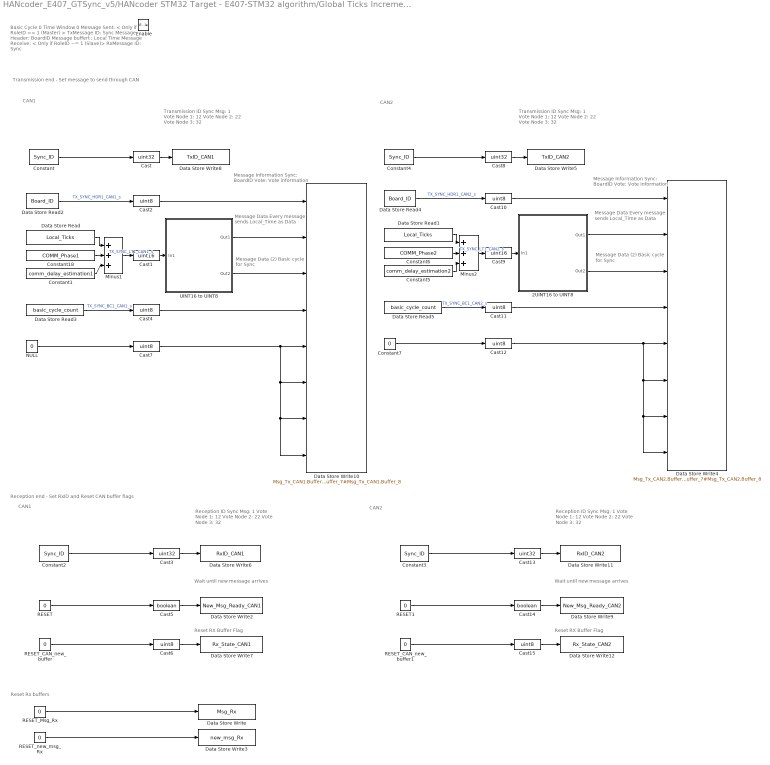
== system HANcoder_E407_GTSync_v5/HANcoder STM32 Target - E407-STM32 algorithm/Global Ticks Increment/CAN Management/Matrix Cycle Manager/COMM Task - Sync BC1/Sync Msg ==
  note: CAN2
  note: CAN1
  note: Transmission end - Set message to send through CAN
  note: CAN2
  note: CAN1
  note: Reception end - Set RxID and Reset CAN buffer flags
  note: Reset Rx buffers
  note: Wait until new message
      | arrives
  note: Message Data (2)
      |    Basic cycle for Sync
  note: Basic Cycle 0
      | Time Window 0
      | Message Sent: < Only if RoleID == 1 (Master) >
      | 	TxMessage ID: Sync
      | 	Message Header: BoardID
      | 	Message buffert : Local Time
      | Message Receive: < Only if RoleID ~= 1 (Slave)>
      | 	RxMessage ID: Sync
  note: Message Data
      |    Every message sends
      |    Local_Time as Data
  note: Transmission ID
      |    Sync Msg: 1
      |    Vote Node 1: 12
      |    Vote Node 2: 22
      |    Vote Node 3: 32
  note: Message Information
      |    Sync: BoardID
      |    Vote: Vote information
  note: Reception ID
      |    Sync Msg: 1
      |    Vote Node 1: 12
      |    Vote Node 2: 22
      |    Vote Node 3: 32
  note: Reset RX Buffer Flag
  note: Message Data (2)
      |    Basic cycle for Sync
  note: Message Data
      |    Every message sends
      |    Local_Time as Data
  note: Transmission ID
      |    Sync Msg: 1
      |    Vote Node 1: 12
      |    Vote Node 2: 22
      |    Vote Node 3: 32
  note: Message Information
      |    Sync: BoardID
      |    Vote: Vote information
  note: Wait until new message
      | arrives
  note: Reception ID
      |    Sync Msg: 1
      |    Vote Node 1: 12
      |    Vote Node 2: 22
      |    Vote Node 3: 32
  note: Reset RX Buffer Flag
  Enable : EnablePort
  2UINT16 to UINT8 : Subsystem
  Cast{,3,8,13} (4 alike) : DataTypeConversion  OutDataTypeStr=uint32
  Cast1 : DataTypeConversion  OutDataTypeStr=uint16
  Cast{2,4,6..7,10..12,15} (8 alike) : DataTypeConversion  OutDataTypeStr=uint8
  Cast14 : DataTypeConversion  OutDataTypeStr=boolean
  Cast5 : DataTypeConversion  OutDataTypeStr=boolean
  Cast9 : DataTypeConversion  OutDataTypeStr=uint16
  Constant{,2..4} (4 alike) : Constant  Value=Sync_ID
  Constant1 : Constant  Value=comm_delay_estimation1
  Constant18 : Constant  Value=COMM_Phase1
  Constant5 : Constant  Value=comm_delay_estimation2
  Constant6 : Constant  Value=COMM_Phase2
  Constant7 : Constant  Value=0  OutDataTypeStr=uint8
  Data Store Read : DataStoreRead  DataStoreName=Local_Ticks
  Data Store Read1 : DataStoreRead  DataStoreName=Local_Ticks
  Data Store Read2 : DataStoreRead  DataStoreName=Board_ID
  Data Store Read3 : DataStoreRead  DataStoreName=basic_cycle_count
  Data Store Read4 : DataStoreRead  DataStoreName=Board_ID
  Data Store Read5 : DataStoreRead  DataStoreName=basic_cycle_count
  Data Store Write : DataStoreWrite  DataStoreName=Msg_Rx
  Data Store Write10 : DataStoreWrite  DataStoreName=Msg_Tx_CAN1  DataStoreElements=Msg_Tx_CAN1.Buffer_1#Msg_Tx_CAN1.Buffer_2#Msg_Tx_CAN1.Buffer_3#Msg_Tx_CAN1.Buffer_4#Msg_Tx_CAN1.Buffer_5#Msg_Tx_CAN1.Buffer_6#Msg_Tx_CAN1.Buffer_7#Msg_Tx_CAN1.Buffer_8
  Data Store Write11 : DataStoreWrite  DataStoreName=RxID_CAN2
  Data Store Write12 : DataStoreWrite  DataStoreName=Rx_State_CAN2
  Data Store Write2 : DataStoreWrite  DataStoreName=New_Msg_Ready_CAN1
  Data Store Write3 : DataStoreWrite  DataStoreName=new_msg_Rx
  Data Store Write4 : DataStoreWrite  DataStoreName=Msg_Tx_CAN2  DataStoreElements=Msg_Tx_CAN2.Buffer_1#Msg_Tx_CAN2.Buffer_2#Msg_Tx_CAN2.Buffer_3#Msg_Tx_CAN2.Buffer_4#Msg_Tx_CAN2.Buffer_5#Msg_Tx_CAN2.Buffer_6#Msg_Tx_CAN2.Buffer_7#Msg_Tx_CAN2.Buffer_8
  Data Store Write5 : DataStoreWrite  DataStoreName=TxID_CAN2
  Data Store Write6 : DataStoreWrite  DataStoreName=RxID_CAN1
  Data Store Write7 : DataStoreWrite  DataStoreName=Rx_State_CAN1
  Data Store Write8 : DataStoreWrite  DataStoreName=TxID_CAN1
  Data Store Write9 : DataStoreWrite  DataStoreName=New_Msg_Ready_CAN2
  Minus1 : Sum  Inputs=+++
  Minus2 : Sum  Inputs=+++
  NULL : Constant  Value=0  OutDataTypeStr=uint8
  RESET : Constant  Value=0
  RESET1 : Constant  Value=0
  RESET_CAN_new_buffer : Constant  Value=0
  RESET_CAN_new_buffer1 : Constant  Value=0
  RESET_Msg_Rx : Constant  Value=0  OutDataTypeStr=Bus: demux_msg_buffer_type
  RESET_new_msg_Rx : Constant  Value=0  OutDataTypeStr=boolean
  UINT16 to UINT8 : Subsystem
  wires:
  Constant18/1 -> Minus1/2
  Minus1/1 -> Cast1/1  "TX_SYNC_LT1_CAN1_s"
  Cast/1 -> Data Store Write8/1
  Data Store Read/1 -> Minus1/1
  Constant/1 -> Cast/1
  Cast3/1 -> Data Store Write6/1
  Constant2/1 -> Cast3/1
  Cast2/1 -> Data Store Write10/1
  Cast4/1 -> Data Store Write10/4
  Data Store Read3/1 -> Cast4/1  "TX_SYNC_BC1_CAN1_s"
  Data Store Read2/1 -> Cast2/1  "TX_SYNC_HDR1_CAN1_s"
  RESET/1 -> Cast5/1
  Cast5/1 -> Data Store Write2/1
  RESET_Msg_Rx/1 -> Data Store Write/1
  RESET_new_msg_Rx/1 -> Data Store Write3/1
  RESET_CAN_new_buffer/1 -> Cast6/1
  Cast6/1 -> Data Store Write7/1
  Constant1/1 -> Minus1/3
  Cast1/1 -> UINT16 to UINT8/1(In1)
  UINT16 to UINT8/2(Out2) -> Data Store Write10/3
  UINT16 to UINT8/1(Out1) -> Data Store Write10/2
  Cast7/1 -> Data Store Write10/8, Data Store Write10/7, Data Store Write10/6, Data Store Write10/5
  NULL/1 -> Cast7/1
  Constant7/1 -> Cast12/1
  Cast12/1 -> Data Store Write4/8, Data Store Write4/7, Data Store Write4/6, Data Store Write4/5
  2UINT16 to UINT8/1(Out1) -> Data Store Write4/2
  2UINT16 to UINT8/2(Out2) -> Data Store Write4/3
  Cast9/1 -> 2UINT16 to UINT8/1(In1)
  Constant5/1 -> Minus2/3
  Data Store Read4/1 -> Cast10/1  "TX_SYNC_HDR1_CAN2_s"
  Data Store Read5/1 -> Cast11/1  "TX_SYNC_BC1_CAN2_s"
  Cast11/1 -> Data Store Write4/4
  Cast10/1 -> Data Store Write4/1
  Constant4/1 -> Cast8/1
  Data Store Read1/1 -> Minus2/1
  Cast8/1 -> Data Store Write5/1
  Minus2/1 -> Cast9/1  "TX_SYNC_LT1_CAN2_s"
  Constant6/1 -> Minus2/2
  Cast15/1 -> Data Store Write12/1
  RESET_CAN_new_buffer1/1 -> Cast15/1
  Cast14/1 -> Data Store Write9/1
  RESET1/1 -> Cast14/1
  Constant3/1 -> Cast13/1
  Cast13/1 -> Data Store Write11/1

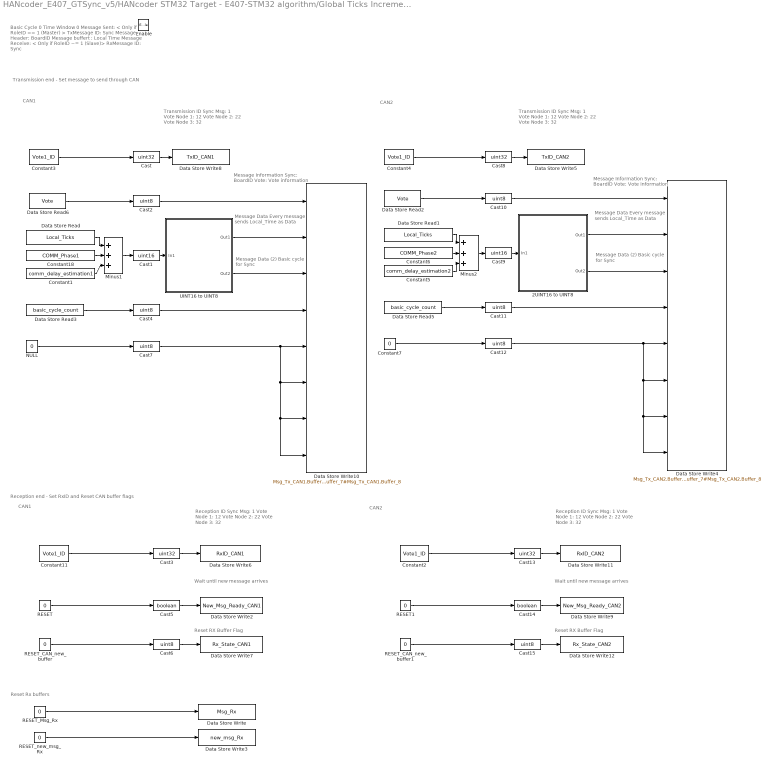
== system HANcoder_E407_GTSync_v5/HANcoder STM32 Target - E407-STM32 algorithm/Global Ticks Increment/CAN Management/Matrix Cycle Manager/COMM Task - Vote1/Vote 1 ==
  note: CAN2
  note: CAN1
  note: Transmission end - Set message to send through CAN
  note: CAN2
  note: CAN1
  note: Reception end - Set RxID and Reset CAN buffer flags
  note: Reset Rx buffers
  note: Wait until new message
      | arrives
  note: Message Data (2)
      |    Basic cycle for Sync
  note: Basic Cycle 0
      | Time Window 0
      | Message Sent: < Only if RoleID == 1 (Master) >
      | 	TxMessage ID: Sync
      | 	Message Header: BoardID
      | 	Message buffert : Local Time
      | Message Receive: < Only if RoleID ~= 1 (Slave)>
      | 	RxMessage ID: Sync
  note: Message Data
      |    Every message sends
      |    Local_Time as Data
  note: Transmission ID
      |    Sync Msg: 1
      |    Vote Node 1: 12
      |    Vote Node 2: 22
      |    Vote Node 3: 32
  note: Message Information
      |    Sync: BoardID
      |    Vote: Vote information
  note: Reception ID
      |    Sync Msg: 1
      |    Vote Node 1: 12
      |    Vote Node 2: 22
      |    Vote Node 3: 32
  note: Reset RX Buffer Flag
  note: Message Data (2)
      |    Basic cycle for Sync
  note: Message Data
      |    Every message sends
      |    Local_Time as Data
  note: Transmission ID
      |    Sync Msg: 1
      |    Vote Node 1: 12
      |    Vote Node 2: 22
      |    Vote Node 3: 32
  note: Message Information
      |    Sync: BoardID
      |    Vote: Vote information
  note: Wait until new message
      | arrives
  note: Reception ID
      |    Sync Msg: 1
      |    Vote Node 1: 12
      |    Vote Node 2: 22
      |    Vote Node 3: 32
  note: Reset RX Buffer Flag
  Enable : EnablePort
  2UINT16 to UINT8 : Subsystem
  Cast{,3,8,13} (4 alike) : DataTypeConversion  OutDataTypeStr=uint32
  Cast1 : DataTypeConversion  OutDataTypeStr=uint16
  Cast{2,4,6..7,10..12,15} (8 alike) : DataTypeConversion  OutDataTypeStr=uint8
  Cast14 : DataTypeConversion  OutDataTypeStr=boolean
  Cast5 : DataTypeConversion  OutDataTypeStr=boolean
  Cast9 : DataTypeConversion  OutDataTypeStr=uint16
  Constant1 : Constant  Value=comm_delay_estimation1
  Constant{2..4,11} (4 alike) : Constant  Value=Vote1_ID
  Constant18 : Constant  Value=COMM_Phase1
  Constant5 : Constant  Value=comm_delay_estimation2
  Constant6 : Constant  Value=COMM_Phase2
  Constant7 : Constant  Value=0  OutDataTypeStr=uint8
  Data Store Read : DataStoreRead  DataStoreName=Local_Ticks
  Data Store Read1 : DataStoreRead  DataStoreName=Local_Ticks
  Data Store Read2 : DataStoreRead  DataStoreName=Vote
  Data Store Read3 : DataStoreRead  DataStoreName=basic_cycle_count
  Data Store Read5 : DataStoreRead  DataStoreName=basic_cycle_count
  Data Store Read6 : DataStoreRead  DataStoreName=Vote
  Data Store Write : DataStoreWrite  DataStoreName=Msg_Rx
  Data Store Write10 : DataStoreWrite  DataStoreName=Msg_Tx_CAN1  DataStoreElements=Msg_Tx_CAN1.Buffer_1#Msg_Tx_CAN1.Buffer_2#Msg_Tx_CAN1.Buffer_3#Msg_Tx_CAN1.Buffer_4#Msg_Tx_CAN1.Buffer_5#Msg_Tx_CAN1.Buffer_6#Msg_Tx_CAN1.Buffer_7#Msg_Tx_CAN1.Buffer_8
  Data Store Write11 : DataStoreWrite  DataStoreName=RxID_CAN2
  Data Store Write12 : DataStoreWrite  DataStoreName=Rx_State_CAN2
  Data Store Write2 : DataStoreWrite  DataStoreName=New_Msg_Ready_CAN1
  Data Store Write3 : DataStoreWrite  DataStoreName=new_msg_Rx
  Data Store Write4 : DataStoreWrite  DataStoreName=Msg_Tx_CAN2  DataStoreElements=Msg_Tx_CAN2.Buffer_1#Msg_Tx_CAN2.Buffer_2#Msg_Tx_CAN2.Buffer_3#Msg_Tx_CAN2.Buffer_4#Msg_Tx_CAN2.Buffer_5#Msg_Tx_CAN2.Buffer_6#Msg_Tx_CAN2.Buffer_7#Msg_Tx_CAN2.Buffer_8
  Data Store Write5 : DataStoreWrite  DataStoreName=TxID_CAN2
  Data Store Write6 : DataStoreWrite  DataStoreName=RxID_CAN1
  Data Store Write7 : DataStoreWrite  DataStoreName=Rx_State_CAN1
  Data Store Write8 : DataStoreWrite  DataStoreName=TxID_CAN1
  Data Store Write9 : DataStoreWrite  DataStoreName=New_Msg_Ready_CAN2
  Minus1 : Sum  Inputs=+++
  Minus2 : Sum  Inputs=+++
  NULL : Constant  Value=0  OutDataTypeStr=uint8
  RESET : Constant  Value=0
  RESET1 : Constant  Value=0
  RESET_CAN_new_buffer : Constant  Value=0
  RESET_CAN_new_buffer1 : Constant  Value=0
  RESET_Msg_Rx : Constant  Value=0  OutDataTypeStr=Bus: demux_msg_buffer_type
  RESET_new_msg_Rx : Constant  Value=0  OutDataTypeStr=boolean
  UINT16 to UINT8 : Subsystem
  wires:
  Constant18/1 -> Minus1/2
  Minus1/1 -> Cast1/1
  Cast/1 -> Data Store Write8/1
  Data Store Read/1 -> Minus1/1
  Constant3/1 -> Cast/1
  Cast3/1 -> Data Store Write6/1
  Constant11/1 -> Cast3/1
  Cast2/1 -> Data Store Write10/1
  Cast4/1 -> Data Store Write10/4
  Data Store Read3/1 -> Cast4/1
  Data Store Read6/1 -> Cast2/1
  RESET/1 -> Cast5/1
  Cast5/1 -> Data Store Write2/1
  RESET_Msg_Rx/1 -> Data Store Write/1
  RESET_new_msg_Rx/1 -> Data Store Write3/1
  RESET_CAN_new_buffer/1 -> Cast6/1
  Cast6/1 -> Data Store Write7/1
  Constant1/1 -> Minus1/3
  Cast1/1 -> UINT16 to UINT8/1(In1)
  UINT16 to UINT8/2(Out2) -> Data Store Write10/3
  UINT16 to UINT8/1(Out1) -> Data Store Write10/2
  Cast7/1 -> Data Store Write10/8, Data Store Write10/7, Data Store Write10/6, Data Store Write10/5
  NULL/1 -> Cast7/1
  Constant7/1 -> Cast12/1
  Cast12/1 -> Data Store Write4/8, Data Store Write4/7, Data Store Write4/6, Data Store Write4/5
  2UINT16 to UINT8/1(Out1) -> Data Store Write4/2
  2UINT16 to UINT8/2(Out2) -> Data Store Write4/3
  Cast9/1 -> 2UINT16 to UINT8/1(In1)
  Constant5/1 -> Minus2/3
  Data Store Read2/1 -> Cast10/1
  Data Store Read5/1 -> Cast11/1
  Cast11/1 -> Data Store Write4/4
  Cast10/1 -> Data Store Write4/1
  Constant4/1 -> Cast8/1
  Data Store Read1/1 -> Minus2/1
  Cast8/1 -> Data Store Write5/1
  Minus2/1 -> Cast9/1
  Constant6/1 -> Minus2/2
  Cast15/1 -> Data Store Write12/1
  RESET_CAN_new_buffer1/1 -> Cast15/1
  Cast14/1 -> Data Store Write9/1
  RESET1/1 -> Cast14/1
  Constant2/1 -> Cast13/1
  Cast13/1 -> Data Store Write11/1
